simulink model "Hyperloop_Levitation_System"  (R2025a)
settings: Solver=VariableStepAuto  StartTime=0.0  StopTime=20  RelTol=1e-3
libraries: slpidlib x1, sharedTrackingLibrary x1
settings Model: Creator=kreenadesai  LastModifiedBy=kreenadesai

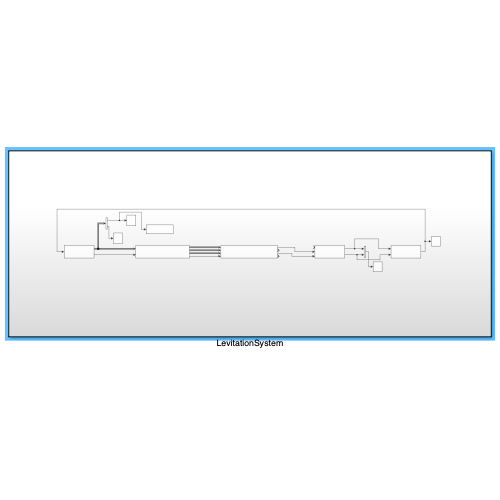
[thumbnail: Simulink's stored preview of the top-level diagram]
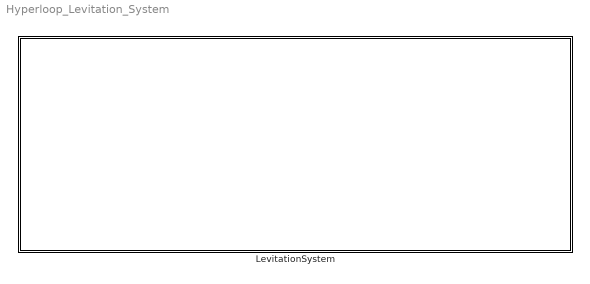
== system Hyperloop_Levitation_System ==
  LevitationSystem : Subsystem

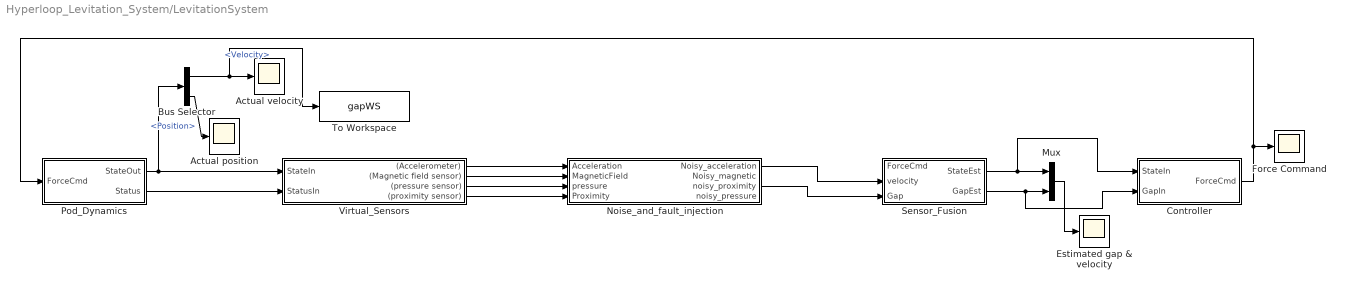
== system Hyperloop_Levitation_System/LevitationSystem ==
  Actual velocity : Scope
      settings: Title=Actual velocity vs Time  ActiveDisplayYMinimum=-0.1  ActiveDisplayYMaximum=0.1  YLabel=Velocity (m/s)  DataLoggingVariableName=ScopeData2
  Actual position : Scope
      settings: Title=Actual position vs Time  ActiveDisplayYMinimum=0  ActiveDisplayYMaximum=0.02  YLabel=pod position (m)  DataLoggingVariableName=ScopeData5
  Bus Selector : BusSelector  OutputSignals=Velocity,Position
  Controller : Subsystem
  Estimated gap & velocity : Scope
      settings: SampleTime=0.001  Title=Sensor Fusion Output Signals  ActiveDisplayYMinimum=-1  ActiveDisplayYMaximum=1  YLabel=Gap and velocity  DataLoggingVariableName=ScopeData3
  Force Command : Scope
      settings: Title=Control Force Command vs Time  ActiveDisplayYMinimum=-7  ActiveDisplayYMaximum=120  YLabel=Control Force (N)  DataLoggingVariableName=ScopeData4
  Mux : Mux  Inputs=2
  Noise_and_fault_injection : Subsystem
  Pod_Dynamics : Subsystem
  Sensor_Fusion : Subsystem
  To Workspace : ToWorkspace  VariableName=gapWS  SaveFormat=Structure With Time  SampleTime=-1
  Virtual_Sensors : Subsystem
  wires:
  Pod_Dynamics/2(Status) -> Virtual_Sensors/2(StatusIn)
  Virtual_Sensors/1((Accelerometer)) -> Noise_and_fault_injection/1(Acceleration)
  Virtual_Sensors/2((Magnetic field sensor)) -> Noise_and_fault_injection/2(MagneticField)
  Noise_and_fault_injection/1(Noisy_acceleration) -> Sensor_Fusion/2(velocity)
  Virtual_Sensors/3((pressure sensor)) -> Noise_and_fault_injection/3(pressure)
  Virtual_Sensors/4((proximity sensor)) -> Noise_and_fault_injection/4(Proximity)
  Noise_and_fault_injection/3(noisy_proximity) -> Sensor_Fusion/3(Gap)
  Pod_Dynamics/1(StateOut) -> Virtual_Sensors/1(StateIn), Bus Selector/1
  Bus Selector/1 -> To Workspace/1, Actual velocity/1  "<Velocity>"
  Controller/1(ForceCmd) -> Force Command/1, Pod_Dynamics/1(ForceCmd)
  Sensor_Fusion/1(StateEst) -> Controller/1(StateIn), Mux/1
  Sensor_Fusion/2(GapEst) -> Controller/2(GapIn), Mux/2
  Mux/1 -> Estimated gap & velocity/1
  Bus Selector/2 -> Actual position/1  "<Position>"

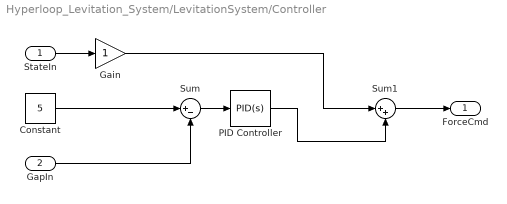
== system Hyperloop_Levitation_System/LevitationSystem/Controller ==
  StateIn : Inport
  GapIn : Inport  Port=2
  Constant : Constant  Value=5
  Gain : Gain
  PID Controller : slpidlib/PID Controller  Controller=PID  Form=Parallel  TimeDomain=Continuous-time  UseExternalTs=off  SampleTime=-1  IntegratorMethod=Forward Euler  FilterMethod=Forward Euler  ControllerParametersSource=internal  P=1  I=1  UseKiTs=off  D=0  UseExternalDerivativeSource=off  N=100  UseFilter=on  TunerSelectOption=Transfer Function Based (PID Tuner App)  InitialConditionSource=internal  InitialConditionForIntegrator=0  InitialConditionForFilter=0  DifferentiatorICPrevScaledInput=0  ExternalReset=none  TrackingMode=off  Kt=1  LimitOutput=off  SatLimitsSource=internal  UpperSaturationLimit=inf  LowerSaturationLimit=-inf  LinearizeAsGain=on  AntiWindupMode=none  Kb=1  LimitIntegrator=off  UpperIntegratorSaturationLimit=inf  LowerIntegratorSaturationLimit=-inf  POutMin=[]  POutMax=[]  IOutMin=[]  IOutMax=[]  DOutMin=[]  DOutMax=[]  NOutMin=[]  NOutMax=[]  SumOutMin=[]  SumOutMax=[]  SaturationOutMin=[]  SaturationOutMax=[]  PParamMin=[]  PParamMax=[]  IParamMin=[]  IParamMax=[]  DParamMin=[]  DParamMax=[]  NParamMin=[]  NParamMax=[]  KbParamMin=[]  KbParamMax=[]  KtParamMin=[]  KtParamMax=[]  KbOutMin=[]  KbOutMax=[]  KtOutMin=[]  KtOutMax=[]  IntegratorOutMin=[]  IntegratorOutMax=[]  FilterOutMin=[]  FilterOutMax=[]  SumI1OutMin=[]  SumI1OutMax=[]  SumI2OutMin=[]  SumI2OutMax=[]  SumI3OutMin=[]  SumI3OutMax=[]  SumI4OutMin=[]  SumI4OutMax=[]  SumDOutMin=[]  SumDOutMax=[]  DifferentiatorOutMin=[]  DifferentiatorOutMax=[]  FilterDiffOutCoefMin=[]  FilterDiffOutCoefMax=[]  ReciprocalOutMin=[]  ReciprocalOutMax=[]  SumDenOutMin=[]  SumDenOutMax=[]  SumNumOutMin=[]  SumNumOutMax=[]  DivideOutMin=[]  DivideOutMax=[]  UdiffTsProdOutMin=[]  UdiffTsProdOutMax=[]  NTsProdOutMin=[]  NTsProdOutMax=[]  UintegralTsProdOutMin=[]  UintegralTsProdOutMax=[]  UngainTsProdOutMin=[]  UngainTsProdOutMax=[]  ClampingZeroOutDataTypeStr=Inherit: Inherit via back propagation  ClampingZeroOutMin=[]  ClampingZeroOutMax=[]  FilterDenConstantOutDataTypeStr=Inherit: Inherit via back propagation  FilterDenConstantOutMin=[]  FilterDenConstantOutMax=[]  PCopyOutDataTypeStr=Inherit: Inherit via back propagation  PCopyOutMin=[]  PCopyOutMax=[]  NCopyOutDataTypeStr=Inherit: Inherit via back propagation  NCopyOutMin=[]  NCopyOutMax=[]  IntegratorContinuousStateAttributes=''  IntegratorStateMustResolveToSignalObject=off  IntegratorRTWStateStorageClass=Auto  FilterContinuousStateAttributes=''  FilterStateMustResolveToSignalObject=off  FilterRTWStateStorageClass=Auto  ParallelPVariant=InternalParameters  IdealPVariant=Disabled  IVariant=InternalParameters  DVariant=InternalParameters  IntegratorVariant=Continuous  SatVariant=Disabled  AWVariant=Passthrough  PCopyVariant=Disabled  TRVariant=Disabled  FdbkBlocksVariant=Forward  IdealPFdbkVariant=Disabled  SatFdbkVariant=Disabled  DerivativeFilterVariant=ContFilter  NVariant=InternalParameters  NCopyVariant=Disabled  FilterICVariant=InternalICsFilter  IntegratorICVariant=InternalICs  ExternalResetVariant=Disabled  TRSumVariant=Passthrough  SumFdbkVariant=Disabled  SumVariant=Sum_PID  TsampFilterVariant=InternalTs  TsampNgainVariant=Passthrough  TsampIntegralVariant=Disabled_SignalSpec  ExternalSaturationOutDataTypeStr=Inherit: Same as second input  DerivativeSourceVariant=ErrorSignal  PreIntVariant=InternalPreInt
  Sum : Sum  Inputs=|+-
  Sum1 : Sum  Inputs=|++
  ForceCmd : Outport
  wires:
  StateIn/1 -> Gain/1
  Constant/1 -> Sum/1
  GapIn/1 -> Sum/2
  Sum/1 -> PID Controller/1
  Gain/1 -> Sum1/1
  PID Controller/1 -> Sum1/2
  Sum1/1 -> ForceCmd/1

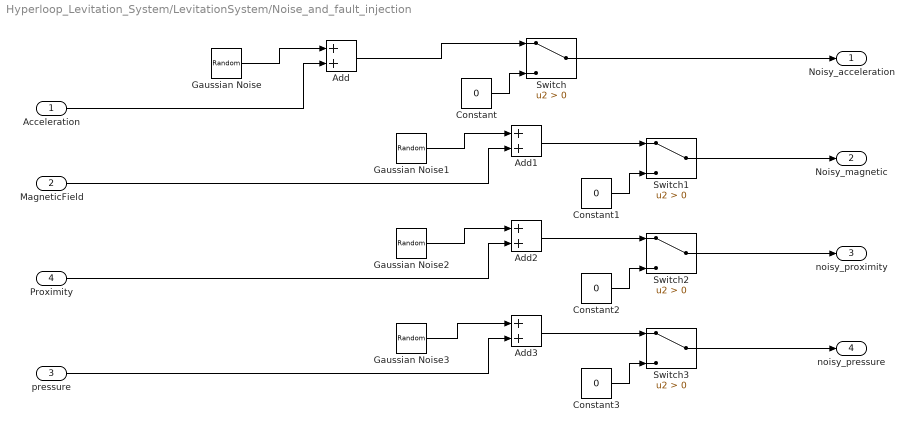
== system Hyperloop_Levitation_System/LevitationSystem/Noise_and_fault_injection ==
  Acceleration : Inport  PortDimensions=1
  MagneticField : Inport  Port=2  PortDimensions=1
  pressure : Inport  Port=3  PortDimensions=1
  Proximity : Inport  Port=4  PortDimensions=1
  Add{,1..3} (4 alike) : Sum
  Constant{,1..3} (4 alike) : Constant  Value=0
  Gaussian Noise : RandomNumber  Variance=0.01  SampleTime=0.1
  Gaussian Noise1 : RandomNumber  Variance=0.05  SampleTime=0.1
  Gaussian Noise2 : RandomNumber  Variance=0.05  SampleTime=0.1
  Gaussian Noise3 : RandomNumber  Variance=0.05  SampleTime=0.1
  Switch{,1..3} (4 alike) : Switch  Criteria=u2 > Threshold  SaturateOnIntegerOverflow=off  InputSameDT=off
  Noisy_acceleration : Outport
  Noisy_magnetic : Outport  Port=2
  noisy_proximity : Outport  Port=3  PortDimensions=1
  noisy_pressure : Outport  Port=4  PortDimensions=1
  wires:
  Gaussian Noise/1 -> Add/1
  Gaussian Noise1/1 -> Add1/1
  Gaussian Noise2/1 -> Add2/1
  Acceleration/1 -> Add/2
  MagneticField/1 -> Add1/2
  Proximity/1 -> Add2/2
  Add/1 -> Switch/1
  Constant/1 -> Switch/3
  Switch/1 -> Noisy_acceleration/1
  Constant1/1 -> Switch1/3
  Add1/1 -> Switch1/1
  Switch1/1 -> Noisy_magnetic/1
  Constant2/1 -> Switch2/3
  Add2/1 -> Switch2/1
  Switch2/1 -> noisy_proximity/1
  Constant3/1 -> Switch3/3
  Switch3/1 -> noisy_pressure/1
  pressure/1 -> Add3/2
  Add3/1 -> Switch3/1
  Gaussian Noise3/1 -> Add3/1

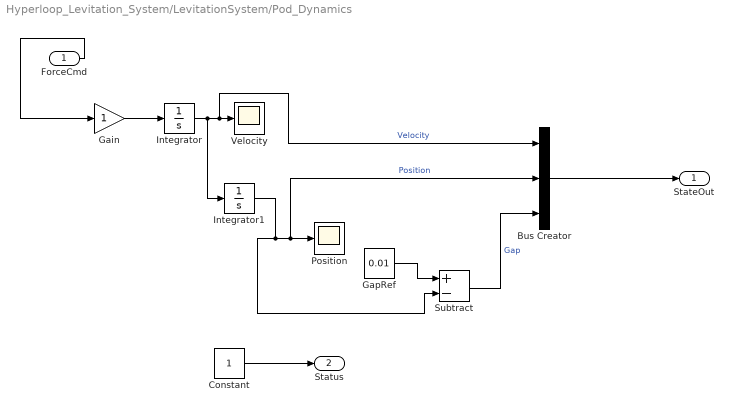
== system Hyperloop_Levitation_System/LevitationSystem/Pod_Dynamics ==
  ForceCmd : Inport
  Bus Creator : BusCreator  Inputs=3
  Constant : Constant
  Gain : Gain
  GapRef : Constant  Value=0.01
  Integrator : Integrator  ContinuousStateAttributes='Velocity'
  Integrator1 : Integrator
  Position : Scope
      settings: ActiveDisplayYMinimum=-1  ActiveDisplayYMaximum=1
  Subtract : Sum  Inputs=+-
  Velocity : Scope
      settings: ActiveDisplayYMinimum=-1  ActiveDisplayYMaximum=1
  StateOut : Outport
  Status : Outport  Port=2
  wires:
  ForceCmd/1 -> Gain/1
  Gain/1 -> Integrator/1
  Integrator/1 -> Bus Creator/1, Velocity/1, Integrator1/1  "Velocity"
  Integrator1/1 -> Bus Creator/2, Position/1, Subtract/2  "Position"
  GapRef/1 -> Subtract/1
  Subtract/1 -> Bus Creator/3  "Gap"
  Constant/1 -> Status/1
  Bus Creator/1 -> StateOut/1

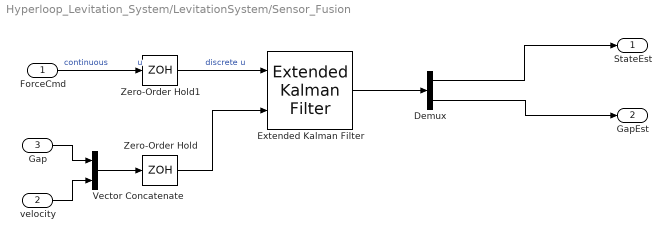
== system Hyperloop_Levitation_System/LevitationSystem/Sensor_Fusion ==
  ForceCmd : Inport
  velocity : Inport  Port=2  PortDimensions=1
  Gap : Inport  Port=3  PortDimensions=1
  Demux : Demux  Outputs=2
  Extended Kalman Filter : sharedTrackingLibrary/Extended Kalman Filter  StateTransitionFcn=myStateTransitionFcn  HasStateTransitionJacobianFcn=off  HasAdditiveProcessNoise=Additive  ProcessNoise=[1e-7 0;0 1e-4]  HasTimeVaryingProcessNoise=off  HasStateTransitionFcnExtraArgument=1  InitialState=[0.0001;0]  InitialStateCovariance=[1e-4 0;0 1e-3]  MeasurementFcn1=myMeasurementFcn  HasMeasurementJacobianFcn1=off  HasMeasurementEnablePort1=off  HasAdditiveMeasurementNoise1=Additive  MeasurementNoise1=[1e-4 0;0 1e-3]  HasTimeVaryingMeasurementNoise1=off  HasMeasurementFcnExtraArgument1=0  HasMeasurementWrapping1=off  MeasurementFcn2=myMeasurementFcn  HasMeasurementJacobianFcn2=off  HasMeasurementEnablePort2=off  HasAdditiveMeasurementNoise2=Additive  MeasurementNoise2=1  HasTimeVaryingMeasurementNoise2=off  HasMeasurementFcnExtraArgument2=0  HasMeasurementWrapping2=off  MeasurementFcn3=myMeasurementFcn  HasMeasurementJacobianFcn3=off  HasMeasurementEnablePort3=off  HasAdditiveMeasurementNoise3=Additive  MeasurementNoise3=1  HasTimeVaryingMeasurementNoise3=off  HasMeasurementFcnExtraArgument3=0  HasMeasurementWrapping3=off  MeasurementFcn4=myMeasurementFcn  HasMeasurementJacobianFcn4=off  HasMeasurementEnablePort4=off  HasAdditiveMeasurementNoise4=Additive  MeasurementNoise4=1  HasTimeVaryingMeasurementNoise4=off  HasMeasurementFcnExtraArgument4=0  HasMeasurementWrapping4=off  MeasurementFcn5=myMeasurementFcn  HasMeasurementJacobianFcn5=off  HasMeasurementEnablePort5=off  HasAdditiveMeasurementNoise5=Additive  MeasurementNoise5=1  HasTimeVaryingMeasurementNoise5=off  HasMeasurementFcnExtraArgument5=0  HasMeasurementWrapping5=off  EnableMultirate=off  StateTransitionFcnSampleTime=1  MeasurementFcn1SampleTime=1  MeasurementFcn2SampleTime=1  MeasurementFcn3SampleTime=1  MeasurementFcn4SampleTime=1  MeasurementFcn5SampleTime=1  UseCurrentEstimator=on  OutputStateCovariance=off  DataType=double  SampleTime=0.001  NumberOfMeasurements=1
  Vector Concatenate : Concatenate
  Zero-Order Hold : ZeroOrderHold  SampleTime=0.001
  Zero-Order Hold1 : ZeroOrderHold  SampleTime=0.001
  StateEst : Outport
  GapEst : Outport  Port=2
  wires:
  Extended Kalman Filter/1 -> Demux/1
  Demux/1 -> StateEst/1
  Demux/2 -> GapEst/1
  Gap/1 -> Vector Concatenate/1
  velocity/1 -> Vector Concatenate/2
  Vector Concatenate/1 -> Zero-Order Hold/1
  Zero-Order Hold/1 -> Extended Kalman Filter/2
  Zero-Order Hold1/1 -> Extended Kalman Filter/1  "discrete u"
  ForceCmd/1 -> Zero-Order Hold1/1  "continuous           u"

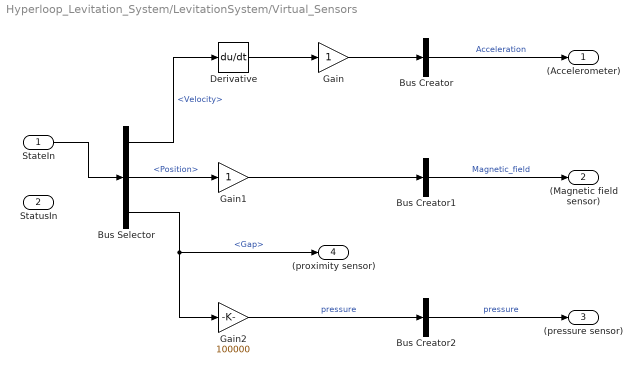
== system Hyperloop_Levitation_System/LevitationSystem/Virtual_Sensors ==
  StateIn : Inport
  StatusIn : Inport  Port=2
  Bus Creator : BusCreator  Inputs=1
  Bus Creator1 : BusCreator  Inputs=1
  Bus Creator2 : BusCreator  Inputs=1
  Bus Selector : BusSelector  OutputSignals=Velocity,Position,Gap
  Derivative : Derivative
  Gain : Gain
  Gain1 : Gain
  Gain2 : Gain  Gain=100000
  (Accelerometer) : Outport
  (Magnetic field sensor) : Outport  Port=2
  (pressure sensor) : Outport  Port=3
  (proximity sensor) : Outport  Port=4
  wires:
  StateIn/1 -> Bus Selector/1
  Bus Selector/1 -> Derivative/1  "<Velocity>"
  Derivative/1 -> Gain/1
  Bus Selector/2 -> Gain1/1  "<Position>"
  Gain/1 -> Bus Creator/1
  Gain1/1 -> Bus Creator1/1
  Bus Creator/1 -> (Accelerometer)/1  "Acceleration"
  Bus Creator1/1 -> (Magnetic field sensor)/1  "Magnetic_field"
  Bus Selector/3 -> Gain2/1, (proximity sensor)/1  "<Gap>"
  Gain2/1 -> Bus Creator2/1  "pressure"
  Bus Creator2/1 -> (pressure sensor)/1  "pressure"
